simulink model "exercise_modelv3"  (R2022a)
settings: Solver=FixedStepAuto  StartTime=0.0  StopTime=Ts  FixedStep=sampling  RelTol=1e-3
values from neighbouring files (symbols this model uses):
  L = 3    [MultiAgent_initiateSAC.m]    (also in control_velocity.m; initiate.m; initiateHybrid.m; initiateSAC.m)
  ld = 5    [MultiAgent_initiateSAC.m]    (also in control_velocity.m; initiate.m; initiateHybrid.m; initiateSAC.m)
  psi_o = 0    [MultiAgent_initiateSAC.m]    (also in control_velocity.m; initiate.m; initiateHybrid.m = thetaRefs(1)*(pi/180); initiateSAC.m)
  sampling = 0.1    [MultiAgent_initiateSAC.m]    (also in control_velocity.m; initiate.m = 0.01; initiateHybrid.m = 0.01; initiateSAC.m)
  Ts = 100    [MultiAgent_initiateSAC.m]    (also in control_velocity.m; initiate.m; initiateHybrid.m = 50; initiateSAC.m)
  vel = 5    [MultiAgent_initiateSAC.m]    (also in control_velocity.m = 7; initiate.m = 10; initiateHybrid.m; initiateSAC.m)
  X_o = refPose(1,1)+0    [MultiAgent_initiateSAC.m]    (also in control_velocity.m; initiate.m = refPose(1,1)+60; initiateHybrid.m = xRef(1); initiateSAC.m)
  xRef = refPose(:,1)    [MultiAgent_initiateSAC.m]    (also in control_velocity.m; initiate.m; initiateHybrid.m; initiateSAC.m)
  xteInt = sqrt((cnormal_xRef(idxc(1))-X_o)^2+(cnormal_yRef(idxc(1))-Y_o)^2)    [MultiAgent_initiateSAC.m]    (also in control_velocity.m; initiate.m; initiateSAC.m; initiateTD3.m)
  Y_o = -refPose(1,2)+20    [MultiAgent_initiateSAC.m]    (also in control_velocity.m = -refPose(1,2)+0; initiate.m; initiateHybrid.m = yRef(1); initiateSAC.m = -refPose(1,2)+0)
  yRef = -refPose(:,2)    [MultiAgent_initiateSAC.m]    (also in control_velocity.m; initiate.m; initiateHybrid.m; initiateSAC.m)
undefined symbols (not defined in the file or in its folder): C_af, C_ar, DiscIntNeverNeededParam, I_z, l_f, l_r, m, psi
libraries: robotalgslib x1, rllib x1
settings Model: Creator=berka  LastModifiedBy=musa
settings DebuggingCC: UnconnectedInputMsg=warning  UnconnectedOutputMsg=warning  UnconnectedLineMsg=warning
settings RTWCC: DLArmComputeVersion=19.05

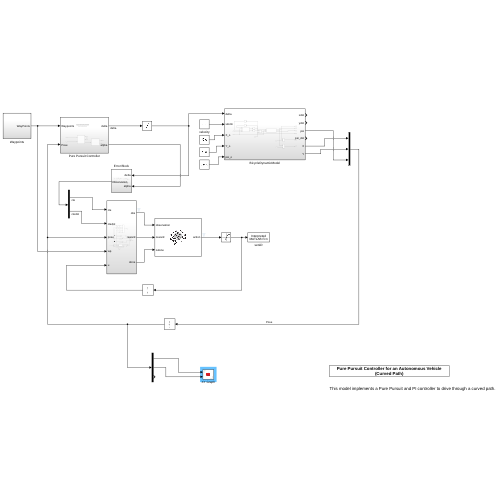
[thumbnail: Simulink's stored preview of the top-level diagram]
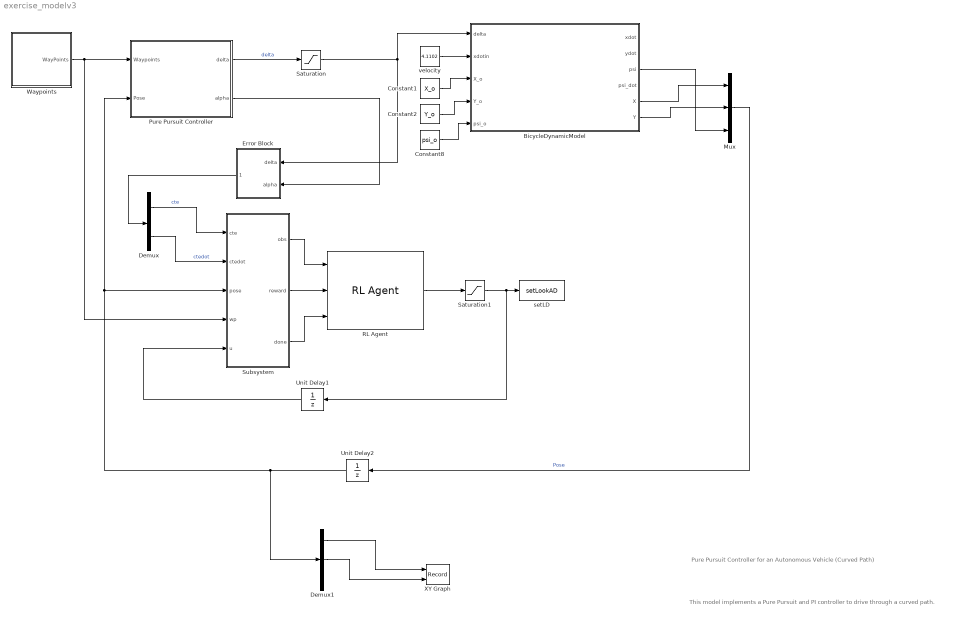
== system exercise_modelv3 ==
  note: This model implements a Pure Pursuit and PI controller to drive through a curved path.
  note: Pure Pursuit Controller for an Autonomous Vehicle
      | (Curved Path)
  "BicycleDynamicModel " : Subsystem
  Constant1 : Constant  Value=X_o
  Constant2 : Constant  Value=Y_o
  Constant8 : Constant  Value=psi_o
  Demux : Demux  Outputs=2
  Demux1 : Demux  Outputs=3
  Error Block : Subsystem
  Mux : Mux  Inputs=3
  Pure Pursuit Controller : Subsystem
  RL Agent : rllib/RL Agent  Agent=agent  ExternalActionAsInput=off  ProvideLastAction=off  ProvideCumRwd=off  TreatAsDirectFeedthrough=on  UseStrictObservationDataTypes=off
  Saturation : Saturate
  Saturation1 : Saturate  UpperLimit=50  LowerLimit=0.5
  Subsystem : Subsystem
  Unit Delay1 : UnitDelay  SampleTime=-1  HasFrameUpgradeWarning=on
  Unit Delay2 : UnitDelay  InitialCondition=[X_o Y_o psi_o]  SampleTime=sampling  HasFrameUpgradeWarning=on
  Waypoints : Subsystem
  XY Graph : Record  FileSettingsInternal="{\"entries\":[{\"content\":{\"excelSettings\":{\"content\":{},\"type\":\"Streamout.ExcelSettings\"}},\"type\":\"Streamout.FileSettingStorage\",\"uuid\":\"67c02c02-4f2d-4f82-a7b6-5958931d64b8\"}],\"packageUris\":[\"http://schema.mathworks.com/mf0/streamout_blocks/R2020a\"],\"version\":\"1.0\"}"  Layout=[1 1]  SignalsInternal="{\"entries\":[{\"content\":{\"signals\":[{\"content\":{\"blockPath\":[\"exercise_modelv3/XY Graph\"],\"channel\":[],\"dimensions\":[1],\"domain\":\"exercise_modelv3/XY Graph\",\"lineColor\":\"#a2142f\",\"plots\":[1],\"port\":1,\"sid\":[\"\"],\"signalID\":26917,\"signalName\":\"Demux1:1\"},\"type\":\"RecordBlkView.Signal\",\"uuid\":\"b8f8e470-a378-49b4-b4d8-d6e230ed7d23\"},{\"content\":{\"blockPath\":[\"exercise_modelv3/XY Graph\"],\"channel\":[],\"dimensions\":[1],\"domain\":\"exercise_modelv3/XY Graph\",\"lineColor\":\"#139fff\",\"plots\":[1],\"port\":2,\"sid\":[\"\"],\"signalID\":26921,\"signalName\":\"Demux1:2\"},\"type\":\"RecordBlkView.Signal\",\"uuid\":\"f1fb7a77-6dad-4636-984f-3bd81f39f1b9\"}]},\"type\":\"RecordBlkView.InputSignals\",\"uuid\":\"fb5c5702-f739-448f-842d-e73fe9f2e07c\"}],\"packageUris\":[\"http://schema.mathworks.com/mf0/streamout_blocks/R2020a\"],\"version\":\"1.0\"}"  VisualizationBindings="{\"xyplotplugin\":{\"info\":[{\"series\":[{\"bindingParametersList\":[{\"parameter\":\"X-Axis\",\"signalID\":26917,\"signalName\":\"Demux1:1\"},{\"parameter\":\"Y-Axis\",\"signalID\":26921,\"signalName\":\"Demux1:2\"}],\"seriesID\":57752}],\"subplotID\":1}]}}"  CompatibilityTag=XY
  setLD : MATLABFcn  MATLABFcn=setLookAD  OutputDimensions=0
  velocity : Constant  Value=4.1102
  wires:
  Waypoints/1(WayPoints) -> Pure Pursuit Controller/1(Waypoints), Subsystem/4(wp)
  Mux/1 -> Unit Delay2/1  "Pose"
  Saturation/1 -> "BicycleDynamicModel "/1(delta), Error Block/1(delta)
  Pure Pursuit Controller/1(delta) -> Saturation/1  "delta"
  Pure Pursuit Controller/2(alpha) -> Error Block/2(alpha)
  Unit Delay1/1 -> Subsystem/5(u)
  Subsystem/1(obs) -> RL Agent/1
  Demux/1 -> Subsystem/1(cte)  "cte"
  Demux/2 -> Subsystem/2(ctedot)  "ctedot"
  Error Block/1(Observation) -> Demux/1
  Subsystem/2(reward) -> RL Agent/2
  Saturation1/1 -> Unit Delay1/1, setLD/1
  Subsystem/3(done) -> RL Agent/3
  RL Agent/1 -> Saturation1/1
  Demux1/1 -> XY Graph/1
  Demux1/2 -> XY Graph/2
  velocity/1 -> "BicycleDynamicModel "/2(xdotin)
  Constant1/1 -> "BicycleDynamicModel "/3(X_o)
  Constant2/1 -> "BicycleDynamicModel "/4(Y_o)
  Constant8/1 -> "BicycleDynamicModel "/5(psi_o)
  "BicycleDynamicModel "/5(X) -> Mux/1
  "BicycleDynamicModel "/6(Y) -> Mux/2
  "BicycleDynamicModel "/3(psi) -> Mux/3
  Unit Delay2/1 -> Demux1/1, Pure Pursuit Controller/2(Pose), Subsystem/3(pose)

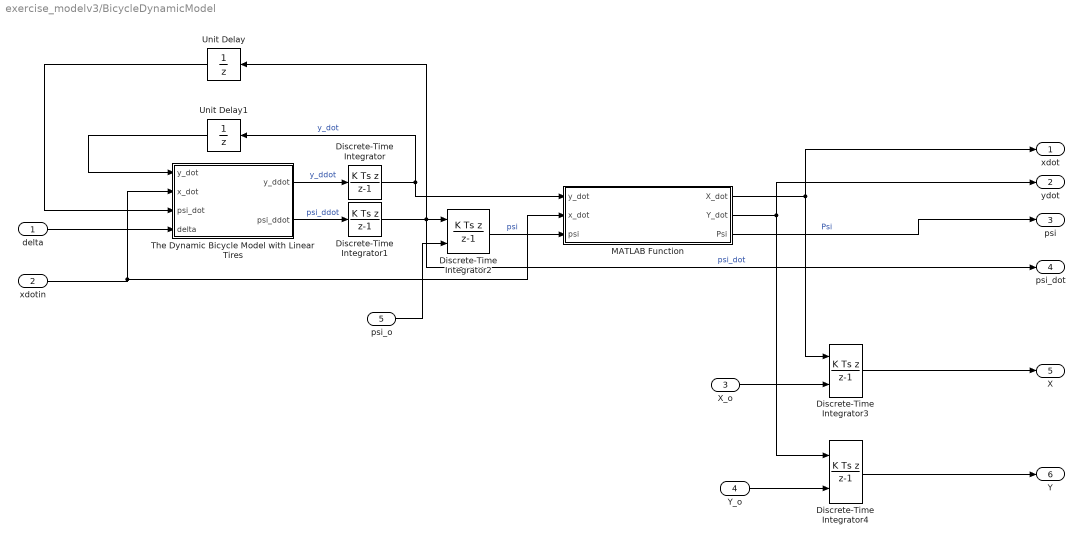
== system exercise_modelv3/BicycleDynamicModel  ==
  delta : Inport
  xdotin : Inport  Port=2
  X_o : Inport  Port=3
  Y_o : Inport  Port=4
  psi_o : Inport  Port=5
  Discrete-Time Integrator : DiscreteIntegrator  IntegratorMethod=Integration: Backward Euler  SampleTime=sampling  ICPrevOutput=DiscIntNeverNeededParam  ICPrevScaledInput=DiscIntNeverNeededParam
  Discrete-Time Integrator1 : DiscreteIntegrator  IntegratorMethod=Integration: Backward Euler  SampleTime=sampling  ICPrevOutput=DiscIntNeverNeededParam  ICPrevScaledInput=DiscIntNeverNeededParam
  Discrete-Time Integrator2 : DiscreteIntegrator  IntegratorMethod=Integration: Backward Euler  InitialConditionSource=external  InitialCondition=psi  SampleTime=sampling  ICPrevOutput=DiscIntNeverNeededParam  ICPrevScaledInput=DiscIntNeverNeededParam
  Discrete-Time Integrator3 : DiscreteIntegrator  IntegratorMethod=Integration: Backward Euler  InitialConditionSource=external  SampleTime=sampling  ICPrevOutput=DiscIntNeverNeededParam  ICPrevScaledInput=DiscIntNeverNeededParam
  Discrete-Time Integrator4 : DiscreteIntegrator  IntegratorMethod=Integration: Backward Euler  InitialConditionSource=external  SampleTime=sampling  ICPrevOutput=DiscIntNeverNeededParam  ICPrevScaledInput=DiscIntNeverNeededParam
  MATLAB Function : MATLAB Function  TreatAsAtomicUnit=on
  The Dynamic Bicycle Model with Linear Tires : Subsystem
  Unit Delay : UnitDelay  SampleTime=-1  HasFrameUpgradeWarning=on
  Unit Delay1 : UnitDelay  SampleTime=-1  HasFrameUpgradeWarning=on
  xdot : Outport
  ydot : Outport  Port=2
  psi : Outport  Port=3
  psi_dot : Outport  Port=4
  X : Outport  Port=5
  Y : Outport  Port=6
  wires:
  delta/1 -> The Dynamic Bicycle Model with Linear Tires/4(delta)
  Discrete-Time Integrator/1 -> Unit Delay1/1, MATLAB Function/1(y_dot)  "y_dot"
  The Dynamic Bicycle Model with Linear Tires/1(y_ddot) -> Discrete-Time Integrator/1  "y_ddot"
  Discrete-Time Integrator1/1 -> psi_dot/1, Unit Delay/1, Discrete-Time Integrator2/1  "psi_dot"
  The Dynamic Bicycle Model with Linear Tires/2(psi_ddot) -> Discrete-Time Integrator1/1  "psi_ddot"
  MATLAB Function/2(Y_dot) -> ydot/1, Discrete-Time Integrator4/1
  Discrete-Time Integrator2/1 -> MATLAB Function/3(psi)  "psi"
  xdotin/1 -> MATLAB Function/2(x_dot), The Dynamic Bicycle Model with Linear Tires/2(x_dot)
  MATLAB Function/3(Psi) -> psi/1  "Psi"
  MATLAB Function/1(X_dot) -> xdot/1, Discrete-Time Integrator3/1
  X_o/1 -> Discrete-Time Integrator3/2
  Discrete-Time Integrator3/1 -> X/1
  Y_o/1 -> Discrete-Time Integrator4/2
  Discrete-Time Integrator4/1 -> Y/1
  psi_o/1 -> Discrete-Time Integrator2/2
  Unit Delay/1 -> The Dynamic Bicycle Model with Linear Tires/3(psi_dot)
  Unit Delay1/1 -> The Dynamic Bicycle Model with Linear Tires/1(y_dot)

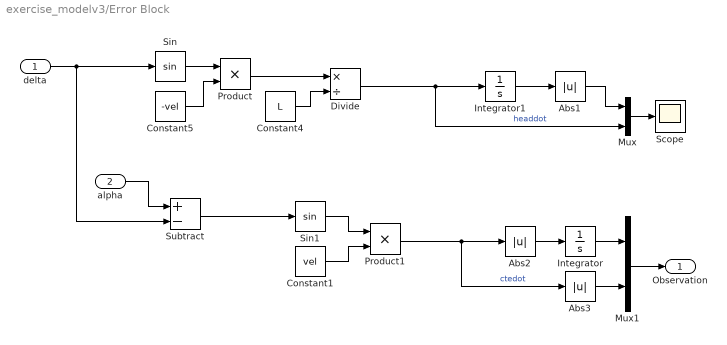
== system exercise_modelv3/Error Block ==
  delta : Inport
  alpha : Inport  Port=2
  Abs1 : Abs  SaturateOnIntegerOverflow=off
  Abs2 : Abs  SaturateOnIntegerOverflow=off
  Abs3 : Abs  SaturateOnIntegerOverflow=off
  Constant1 : Constant  Value=vel
  Constant4 : Constant  Value=L
  Constant5 : Constant  Value=-vel
  Divide : Product  Inputs=*/
  Integrator : Integrator  InitialCondition=xteInt
  Integrator1 : Integrator
  Mux : Mux  Inputs=2
  Mux1 : Mux  Inputs=2
  Product : Product
  Product1 : Product
  Scope : Scope
  Sin : Trigonometry
  Sin1 : Trigonometry
  Subtract : Sum  Inputs=+-
  Observation : Outport
  wires:
  Constant4/1 -> Divide/2
  Sin/1 -> Product/1
  Product/1 -> Divide/1
  delta/1 -> Subtract/2, Sin/1
  Constant5/1 -> Product/2
  Sin1/1 -> Product1/1
  Constant1/1 -> Product1/2
  Subtract/1 -> Sin1/1
  alpha/1 -> Subtract/1
  Divide/1 -> Integrator1/1, Mux/2  "headdot"
  Product1/1 -> Abs3/1, Abs2/1  "ctedot"
  Integrator1/1 -> Abs1/1
  Abs1/1 -> Mux/1
  Mux/1 -> Scope/1
  Mux1/1 -> Observation/1
  Integrator/1 -> Mux1/1
  Abs3/1 -> Mux1/2
  Abs2/1 -> Integrator/1

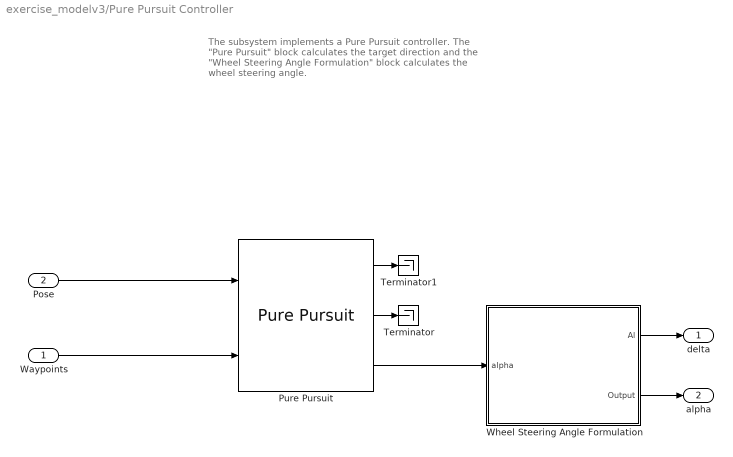
== system exercise_modelv3/Pure Pursuit Controller ==
  note: The subsystem implements a Pure Pursuit controller. The "Pure Pursuit" block calculates the target direction and the "Wheel Steering Angle Formulation" block calculates the wheel steering angle.
  Waypoints : Inport
  Pose : Inport  Port=2
  Pure Pursuit : robotalgslib/Pure Pursuit  DesiredLinearVelocity=4.1102  MaxAngularVelocity=1.0  LookaheadDistance=0.5855  TargetDirPort=on  SimulateUsing=Code generation
  Terminator : Terminator
  Terminator1 : Terminator
  Wheel Steering Angle Formulation : Subsystem  mask{L=L, ld=ld}
      mask prompts: L "Bicycle length"; ld "Lookahead distance"
      mask TypeOptions L: Bicycle length/Value
      mask TypeOptions ld: Lookahead distance/Value
      mask Display:
      | image("GeometryMask.png")
      | port_label('input', 1, 'alpha')
      | port_label('output', 1, 'delta')
  delta : Outport
  alpha : Outport  Port=2
  wires:
  Pure Pursuit/3 -> Wheel Steering Angle Formulation/1(alpha)
  Waypoints/1 -> Pure Pursuit/2
  Pose/1 -> Pure Pursuit/1
  Pure Pursuit/1 -> Terminator1/1
  Pure Pursuit/2 -> Terminator/1
  Wheel Steering Angle Formulation/1(Al) -> delta/1
  Wheel Steering Angle Formulation/2(Output) -> alpha/1

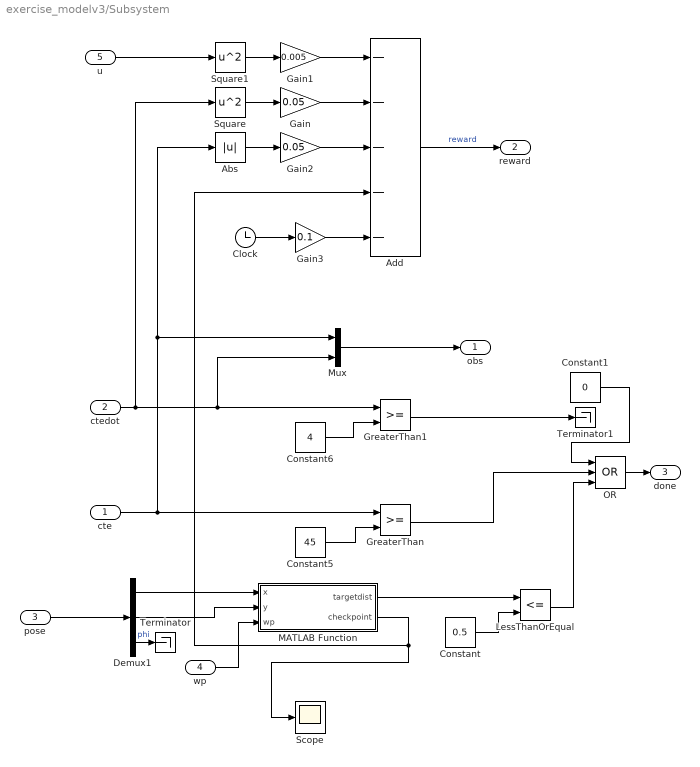
== system exercise_modelv3/Subsystem ==
  cte : Inport
  ctedot : Inport  Port=2
  pose : Inport  Port=3
  wp : Inport  Port=4
  u : Inport  Port=5
  Abs : Abs  SaturateOnIntegerOverflow=off
  Add : Sum  Inputs=-----
  Clock : Clock
  Constant : Constant  Value=0.5
  Constant1 : Constant  Value=0
  Constant5 : Constant  Value=45
  Constant6 : Constant  Value=4
  Demux1 : Demux  Outputs=3
  Gain : Gain  Gain=0.05
  Gain1 : Gain  Gain=0.005
  Gain2 : Gain  Gain=0.05
  Gain3 : Gain  Gain=0.1
  GreaterThan : RelationalOperator  OutDataTypeStr=boolean  RndMeth=Simplest  InputSameDT=off
  GreaterThan1 : RelationalOperator  OutDataTypeStr=boolean  RndMeth=Simplest  InputSameDT=off
  LessThanOrEqual : RelationalOperator  Operator=<=  OutDataTypeStr=boolean  RndMeth=Simplest  InputSameDT=off
  MATLAB Function : MATLAB Function  TreatAsAtomicUnit=on
  Mux : Mux  Inputs=2
  OR : Logic  Operator=OR  Inputs=3  IconShape=distinctive  AllPortsSameDT=off  OutDataTypeStr=boolean
  Scope : Scope
  Square : Math  Operator=square
  Square1 : Math  Operator=square
  Terminator : Terminator
  Terminator1 : Terminator
  obs : Outport
  reward : Outport  Port=2
  done : Outport  Port=3
  wires:
  Constant5/1 -> GreaterThan/2
  Constant6/1 -> GreaterThan1/2
  GreaterThan/1 -> OR/2
  GreaterThan1/1 -> Terminator1/1
  Mux/1 -> obs/1
  Constant/1 -> LessThanOrEqual/2
  Demux1/2 -> MATLAB Function/2(y)
  Demux1/1 -> MATLAB Function/1(x)
  MATLAB Function/1(targetdist) -> LessThanOrEqual/1
  pose/1 -> Demux1/1
  Demux1/3 -> Terminator/1  "phi"
  wp/1 -> MATLAB Function/3(wp)
  cte/1 -> Mux/1, Abs/1, GreaterThan/1
  Abs/1 -> Gain2/1
  Square1/1 -> Gain1/1
  Gain/1 -> Add/2
  Gain1/1 -> Add/1
  ctedot/1 -> Square/1, GreaterThan1/1, Mux/2
  Square/1 -> Gain/1
  u/1 -> Square1/1
  Add/1 -> reward/1  "reward"
  Gain2/1 -> Add/3
  MATLAB Function/2(checkpoint) -> Scope/1, Add/4
  OR/1 -> done/1
  LessThanOrEqual/1 -> OR/3
  Constant1/1 -> OR/1
  Gain3/1 -> Add/5
  Clock/1 -> Gain3/1

== system exercise_modelv3/Waypoints ==
  Constant3 : Constant  Value=xRef  SampleTime=0.1
  Constant4 : Constant  Value=yRef  SampleTime=0.1
  Matrix Concatenate : Concatenate  Mode=Multidimensional array  ConcatenateDimension=2
  WayPoints : Outport
  wires:
  Constant4/1 -> Matrix Concatenate/2
  Matrix Concatenate/1 -> WayPoints/1
  Constant3/1 -> Matrix Concatenate/1

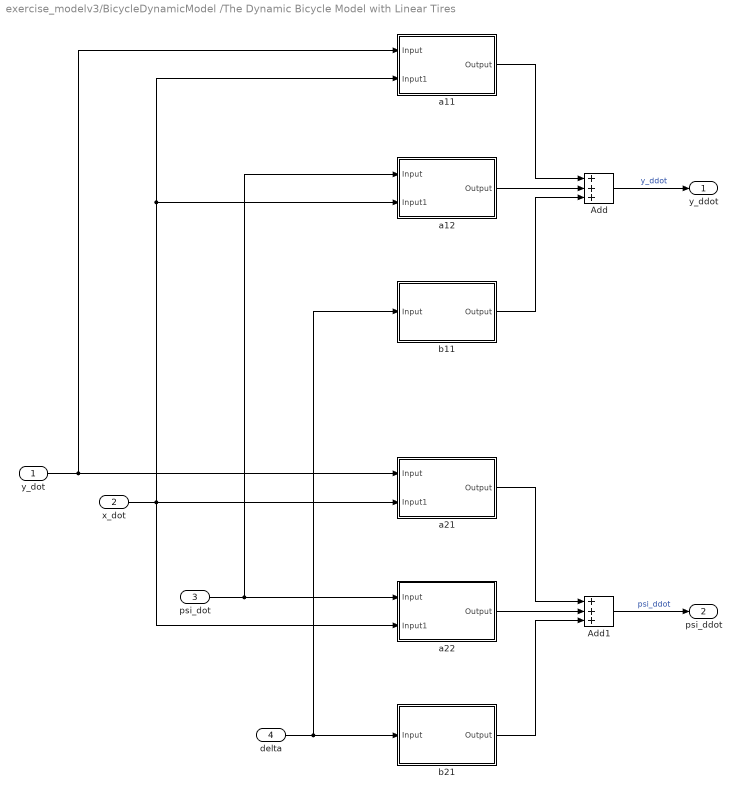
== system exercise_modelv3/BicycleDynamicModel /The Dynamic Bicycle Model with Linear Tires ==
  y_dot : Inport
  x_dot : Inport  Port=2
  psi_dot : Inport  Port=3
  delta : Inport  Port=4
  Add : Sum  Inputs=+++
  Add1 : Sum  Inputs=+++
  a11 : Subsystem
  a12 : Subsystem
  a21 : Subsystem
  a22 : Subsystem
  b11 : Subsystem
  b21 : Subsystem
  y_ddot : Outport
  psi_ddot : Outport  Port=2
  wires:
  b11/1(Output) -> Add/3
  a21/1(Output) -> Add1/1
  a12/1(Output) -> Add/2
  Add1/1 -> psi_ddot/1  "psi_ddot"
  psi_dot/1 -> a22/1(Input), a12/1(Input)
  x_dot/1 -> a22/2(Input1), a21/2(Input1), a11/2(Input1), a12/2(Input1)
  Add/1 -> y_ddot/1  "y_ddot"
  a22/1(Output) -> Add1/2
  b21/1(Output) -> Add1/3
  a11/1(Output) -> Add/1
  delta/1 -> b11/1(Input), b21/1(Input)
  y_dot/1 -> a11/1(Input), a21/1(Input)

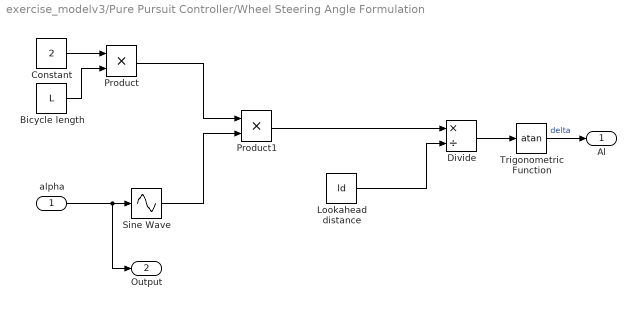
== system exercise_modelv3/Pure Pursuit Controller/Wheel Steering Angle Formulation ==
  alpha : Inport
  Bicycle length : Constant  Value=L
  Constant : Constant  Value=2
  Divide : Product  Inputs=*/
  Lookahead distance : Constant  Value=ld  SampleTime=sampling
  Product : Product
  Product1 : Product
  Sine Wave : Sin  TimeSource=Use external signal  SampleTime=0
  Trigonometric Function : Trigonometry  Operator=atan
  Al : Outport
  Output : Outport  Port=2
  wires:
  Sine Wave/1 -> Product1/2
  Bicycle length/1 -> Product/2
  Constant/1 -> Product/1
  Product1/1 -> Divide/1
  Product/1 -> Product1/1
  Divide/1 -> Trigonometric Function/1
  Trigonometric Function/1 -> Al/1  "delta"
  alpha/1 -> Output/1, Sine Wave/1
  Lookahead distance/1 -> Divide/2

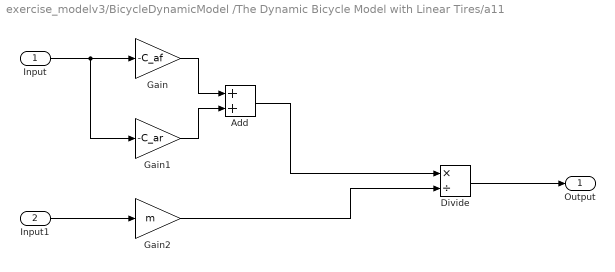
== system exercise_modelv3/BicycleDynamicModel /The Dynamic Bicycle Model with Linear Tires/a11 ==
  Input : Inport
  Input1 : Inport  Port=2
  Add : Sum
  Divide : Product  Inputs=*/
  Gain : Gain  Gain=-C_af
  Gain1 : Gain  Gain=-C_ar
  Gain2 : Gain  Gain=m
  Output : Outport
  wires:
  Input1/1 -> Gain2/1
  Input/1 -> Gain1/1, Gain/1
  Gain/1 -> Add/1
  Divide/1 -> Output/1
  Add/1 -> Divide/1
  Gain1/1 -> Add/2
  Gain2/1 -> Divide/2

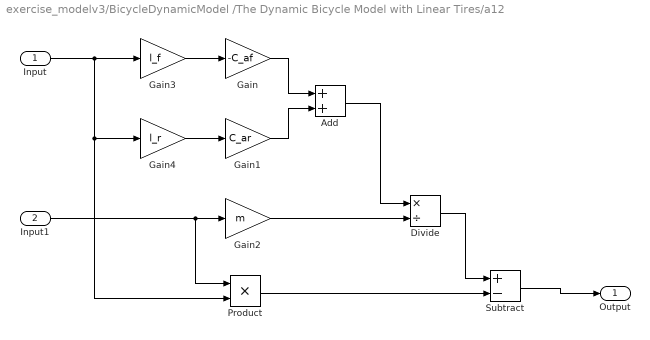
== system exercise_modelv3/BicycleDynamicModel /The Dynamic Bicycle Model with Linear Tires/a12 ==
  Input : Inport
  Input1 : Inport  Port=2
  Add : Sum
  Divide : Product  Inputs=*/
  Gain : Gain  Gain=-C_af
  Gain1 : Gain  Gain=C_ar
  Gain2 : Gain  Gain=m
  Gain3 : Gain  Gain=l_f
  Gain4 : Gain  Gain=l_r
  Product : Product
  Subtract : Sum  Inputs=+-
  Output : Outport
  wires:
  Gain1/1 -> Add/2
  Add/1 -> Divide/1
  Gain2/1 -> Divide/2
  Gain/1 -> Add/1
  Input/1 -> Gain3/1, Product/2, Gain4/1
  Input1/1 -> Product/1, Gain2/1
  Gain3/1 -> Gain/1
  Gain4/1 -> Gain1/1
  Divide/1 -> Subtract/1
  Subtract/1 -> Output/1
  Product/1 -> Subtract/2

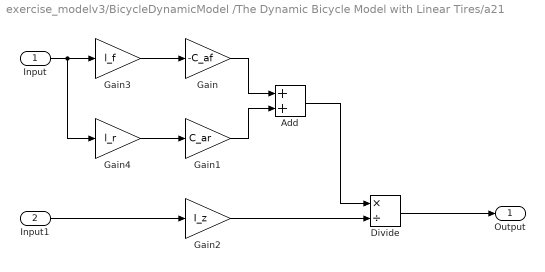
== system exercise_modelv3/BicycleDynamicModel /The Dynamic Bicycle Model with Linear Tires/a21 ==
  Input : Inport
  Input1 : Inport  Port=2
  Add : Sum
  Divide : Product  Inputs=*/
  Gain : Gain  Gain=-C_af
  Gain1 : Gain  Gain=C_ar
  Gain2 : Gain  Gain=I_z
  Gain3 : Gain  Gain=l_f
  Gain4 : Gain  Gain=l_r
  Output : Outport
  wires:
  Input1/1 -> Gain2/1
  Input/1 -> Gain3/1, Gain4/1
  Gain/1 -> Add/1
  Divide/1 -> Output/1
  Gain2/1 -> Divide/2
  Add/1 -> Divide/1
  Gain1/1 -> Add/2
  Gain3/1 -> Gain/1
  Gain4/1 -> Gain1/1

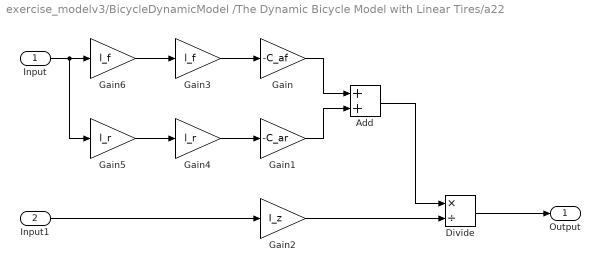
== system exercise_modelv3/BicycleDynamicModel /The Dynamic Bicycle Model with Linear Tires/a22 ==
  Input : Inport
  Input1 : Inport  Port=2
  Add : Sum
  Divide : Product  Inputs=*/
  Gain : Gain  Gain=-C_af
  Gain1 : Gain  Gain=-C_ar
  Gain2 : Gain  Gain=I_z
  Gain3 : Gain  Gain=l_f
  Gain4 : Gain  Gain=l_r
  Gain5 : Gain  Gain=l_r
  Gain6 : Gain  Gain=l_f
  Output : Outport
  wires:
  Gain1/1 -> Add/2
  Add/1 -> Divide/1
  Gain2/1 -> Divide/2
  Gain/1 -> Add/1
  Input/1 -> Gain6/1, Gain5/1
  Input1/1 -> Gain2/1
  Gain3/1 -> Gain/1
  Gain4/1 -> Gain1/1
  Gain5/1 -> Gain4/1
  Gain6/1 -> Gain3/1
  Divide/1 -> Output/1

== system exercise_modelv3/BicycleDynamicModel /The Dynamic Bicycle Model with Linear Tires/b11 ==
  Input : Inport
  Constant : Constant  Value=m  SampleTime=Ts
  Divide : Product  Inputs=*/
  Gain : Gain  Gain=C_af
  Output : Outport
  wires:
  Input/1 -> Gain/1
  Gain/1 -> Divide/1
  Divide/1 -> Output/1
  Constant/1 -> Divide/2

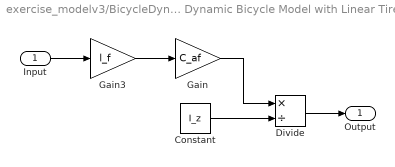
== system exercise_modelv3/BicycleDynamicModel /The Dynamic Bicycle Model with Linear Tires/b21 ==
  Input : Inport
  Constant : Constant  Value=I_z  SampleTime=Ts
  Divide : Product  Inputs=*/
  Gain : Gain  Gain=C_af
  Gain3 : Gain  Gain=l_f
  Output : Outport
  wires:
  Gain3/1 -> Gain/1
  Input/1 -> Gain3/1
  Gain/1 -> Divide/1
  Divide/1 -> Output/1
  Constant/1 -> Divide/2

== matlab function exercise_modelv3/BicycleDynamicModel /MATLAB Function ==
  data: y_dot input; X_dot output; x_dot input; psi input; Y_dot output; Psi output
function [X_dot, Y_dot, Psi]= VehicleCoordinateTransformator(y_dot, x_dot, psi)

Y_dot = x_dot*sin(psi)+y_dot*cos(psi);
X_dot = x_dot*cos(psi)-y_dot*sin(psi);
Psi   = psi;

end

== matlab function exercise_modelv3/Subsystem/MATLAB Function ==
  data: x input; targetdist output; y input; wp input; checkpoint output
function [targetdist, checkpoint] = fcn(x,y,wp)

x_last = wp(end,1);
y_last = wp(end,2);
targetdist = sqrt((x_last-x)^2 + (y_last-y)^2);

checkpoint = 0;

end
